simulink model "DCmotor_EMD4ETI22_Simulink_baseModel_lecture19_PEC"  (R2022a)
settings: Solver=FixedStepAuto  StartTime=0.0  StopTime=15  FixedStep=0.001  RelTol=1e-3
values from neighbouring files (symbols this model uses):
  i0 = 0    [DCmotor_InputData_baseModel_lecture19.m]    (also in DCmotor_InputData_baseModel_lecture19_PEC.m; DCmotor_InputData_baseModel_lecture19_PEC_Supply.m)
  Jeq = Inertia + Inertia_Load    [DCmotor_InputData_baseModel_lecture19.m]    (also in DCmotor_InputData_baseModel_lecture19_PEC.m = 2 * J; DCmotor_InputData_baseModel_lecture19_PEC_Supply.m = 2 * J; DCmotor_TransferFunctions_baseModel_lecture19.m)
  k_d = 0    [DCmotor_InputData_baseModel_lecture19.m]    (also in DCmotor_InputData_baseModel_lecture19_PEC.m = ViscousDamping; DCmotor_InputData_baseModel_lecture19_PEC_Supply.m = ViscousDamping; DCmotor_TransferFunctions_baseModel_lecture19.m)
  kE = Data{11, 5 + 3 * (motorID-1)}    [DCmotor_InputData_baseModel_lecture19.m]    (also in DCmotor_InputData_baseModel_lecture19_PEC.m; DCmotor_InputData_baseModel_lecture19_PEC_Supply.m; DCmotor_TransferFunctions_baseModel_lecture19.m)
  kT = Data{12, 5 + 3 * (motorID-1)}    [DCmotor_InputData_baseModel_lecture19.m]    (also in DCmotor_InputData_baseModel_lecture19_PEC.m = kE; DCmotor_InputData_baseModel_lecture19_PEC_Supply.m = kE; DCmotor_TransferFunctions_baseModel_lecture19.m)
  La = La * 10^-3    [DCmotor_InputData_baseModel_lecture19.m]    (also in DCmotor_InputData_baseModel_lecture19_PEC.m; DCmotor_InputData_baseModel_lecture19_PEC_Supply.m; DCmotor_TransferFunctions_baseModel_lecture19.m)
  pos0 = 0    [DCmotor_InputData_baseModel_lecture19.m]    (also in DCmotor_InputData_baseModel_lecture19_PEC.m; DCmotor_InputData_baseModel_lecture19_PEC_Supply.m)
  Ra_20 = Ra    [DCmotor_InputData_baseModel_lecture19.m]    (also in DCmotor_InputData_baseModel_lecture19_PEC.m; DCmotor_InputData_baseModel_lecture19_PEC_Supply.m; DCmotor_TransferFunctions_baseModel_lecture19.m)
  T_triang = 1/f_triang    (= 0.0002)    [DCmotor_InputData_baseModel_lecture19_PEC.m]    (also in DCmotor_InputData_baseModel_lecture19_PEC_Supply.m)
  V_DC = 1.5 * Voltage    [DCmotor_InputData_baseModel_lecture19_PEC.m]    (also in DCmotor_InputData_baseModel_lecture19_PEC_Supply.m)
  Voltage = Data{5, 5 + 3 * (motorID-1)}    [DCmotor_InputData_baseModel_lecture19.m]    (also in DCmotor_InputData_baseModel_lecture19_PEC.m; DCmotor_InputData_baseModel_lecture19_PEC_Supply.m; DCmotor_TransferFunctions_baseModel_lecture19.m)
  w0 = 0    [DCmotor_InputData_baseModel_lecture19.m]    (also in DCmotor_InputData_baseModel_lecture19_PEC.m; DCmotor_InputData_baseModel_lecture19_PEC_Supply.m)
libraries: simulink x1
settings Model: Creator=lucap  LastModifiedBy=lucap

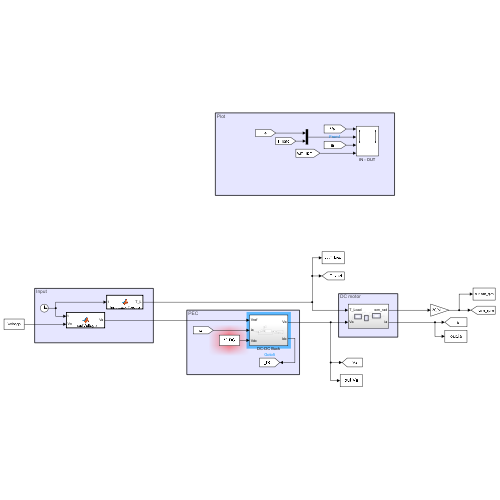
[thumbnail: Simulink's stored preview of the top-level diagram]
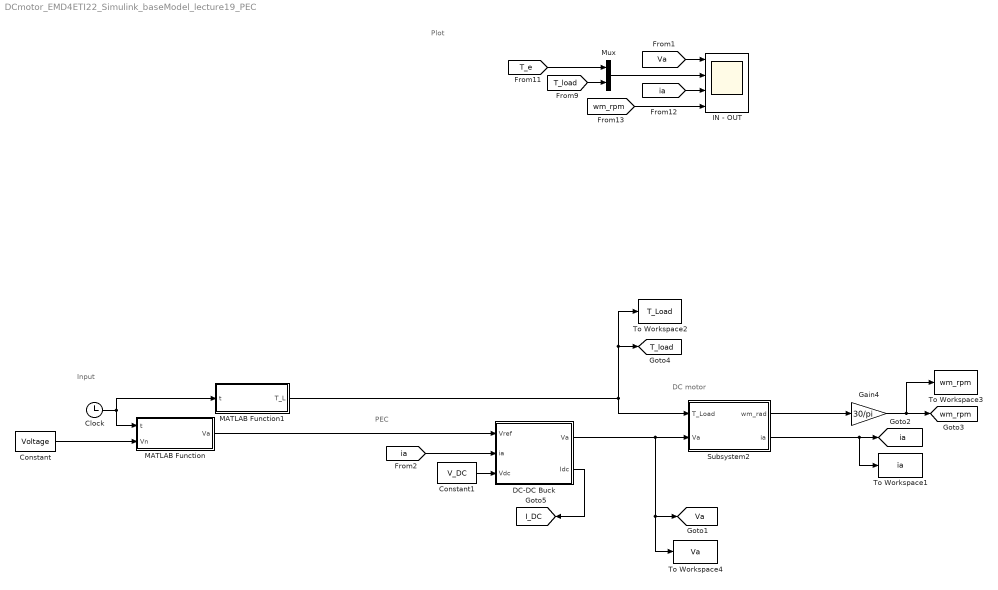
== system DCmotor_EMD4ETI22_Simulink_baseModel_lecture19_PEC ==
  note: PEC
  note: DC motor
  note: Plot
  note: Input
  Clock : Clock
  Constant : Constant  Value=Voltage
  Constant1 : Constant  Value=V_DC
  DC-DC Buck : Subsystem
  Gain4 : Gain  Gain=30/pi
  IN - OUT : Scope  NumInputPorts=4
  MATLAB Function : MATLAB Function  TreatAsAtomicUnit=on
  MATLAB Function1 : MATLAB Function  TreatAsAtomicUnit=on
  Mux : Mux  Inputs=2
  Subsystem2 : Subsystem
  To Workspace1 : ToWorkspace  VariableName=ia  SaveFormat=Structure With Time  SampleTime=-1
  To Workspace2 : ToWorkspace  VariableName=T_Load  SaveFormat=Structure With Time  SampleTime=-1
  To Workspace3 : ToWorkspace  VariableName=wm_rpm  SaveFormat=Structure With Time  SampleTime=-1
  To Workspace4 : ToWorkspace  VariableName=Va  SaveFormat=Structure With Time  SampleTime=-1
  tag scope: I_DC=global, T_load=global, Va=global, ia=global, wm_rpm=global
  wires:
  Subsystem2/1(wm_rad) -> Gain4/1
  Clock/1 -> MATLAB Function/1(t), MATLAB Function1/1(t)
  [T_e] -> Mux/1
  MATLAB Function1/1(T_L) -> [T_load], To Workspace2/1, Subsystem2/1(T_Load)
  Subsystem2/2(ia) -> To Workspace1/1, [ia]
  Gain4/1 -> To Workspace3/1, [wm_rpm]
  [T_load] -> Mux/2
  [Va] -> IN - OUT/1
  [wm_rpm] -> IN - OUT/4
  Constant/1 -> MATLAB Function/2(Vn)
  Mux/1 -> IN - OUT/2
  [ia] -> IN - OUT/3
  DC-DC Buck/1(Va) -> To Workspace4/1, [Va], Subsystem2/2(Va)
  MATLAB Function/1(Va) -> DC-DC Buck/1(Vref)
  [ia] -> DC-DC Buck/2(ia)
  Constant1/1 -> DC-DC Buck/3(Vdc)
  DC-DC Buck/2(Idc) -> [I_DC]

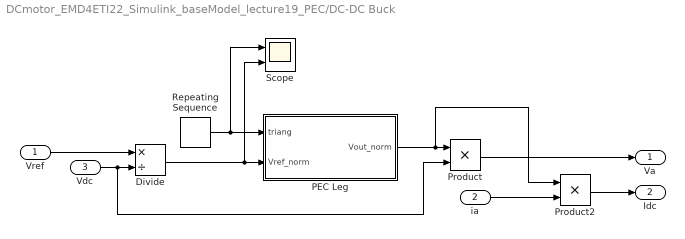
== system DCmotor_EMD4ETI22_Simulink_baseModel_lecture19_PEC/DC-DC Buck ==
  Vref : Inport
  ia : Inport  Port=2
  Vdc : Inport  Port=3
  Divide : Product  Inputs=*/
  PEC Leg : MATLAB Function  TreatAsAtomicUnit=on
  Product : Product
  Product2 : Product
  Repeating Sequence : simulink/Sources/Repeating Sequence  rep_seq_t=[0 T_triang/2 T_triang]  rep_seq_y=[0 1 0]
  Scope : Scope  NumInputPorts=2
  Va : Outport
  Idc : Outport  Port=2
  wires:
  ia/1 -> Product2/2
  Product/1 -> Va/1
  Product2/1 -> Idc/1
  Repeating Sequence/1 -> Scope/1, PEC Leg/1(triang)
  Divide/1 -> Scope/2, PEC Leg/2(Vref_norm)
  Vref/1 -> Divide/1
  Vdc/1 -> Product/2, Divide/2
  PEC Leg/1(Vout_norm) -> Product2/1, Product/1

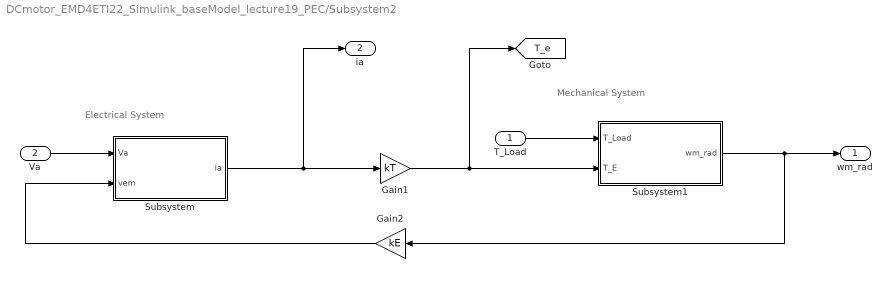
== system DCmotor_EMD4ETI22_Simulink_baseModel_lecture19_PEC/Subsystem2 ==
  note: Mechanical System
  note: Electrical System
  T_Load : Inport
  Va : Inport  Port=2
  Gain1 : Gain  Gain=kT
  Gain2 : Gain  Gain=kE
  Subsystem : Subsystem
  Subsystem1 : Subsystem
  wm_rad : Outport
  ia : Outport  Port=2
  tag scope: T_e=global
  wires:
  Subsystem/1(ia) -> Gain1/1, ia/1
  Subsystem1/1(wm_rad) -> wm_rad/1, Gain2/1
  Gain2/1 -> Subsystem/2(vem)
  Va/1 -> Subsystem/1(Va)
  Gain1/1 -> Subsystem1/2(T_E), [T_e]
  T_Load/1 -> Subsystem1/1(T_Load)

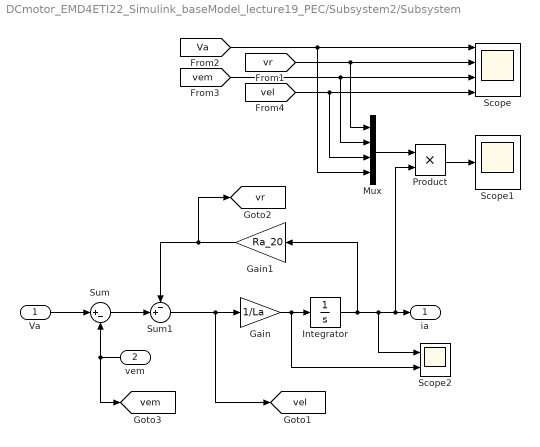
== system DCmotor_EMD4ETI22_Simulink_baseModel_lecture19_PEC/Subsystem2/Subsystem ==
  Va : Inport
  vem : Inport  Port=2
  Gain : Gain  Gain=1/La
  Gain1 : Gain  Gain=Ra_20
  Integrator : Integrator  InitialCondition=i0
  Mux : Mux
  Product : Product
  Scope : Scope  NumInputPorts=4
  Scope1 : Scope
  Scope2 : Scope  NumInputPorts=2
  Sum : Sum  Inputs=|+-
  Sum1 : Sum  Inputs=-+|
  ia : Outport
  tag scope: vel=global, vem=global, vr=global
  wires:
  Gain/1 -> Scope2/2, Integrator/1
  Va/1 -> Sum/1
  Sum/1 -> Sum1/2
  Sum1/1 -> [vel], Gain/1
  Integrator/1 -> Gain1/1, Scope2/1, Product/2, ia/1
  vem/1 -> [vem], Sum/2
  Gain1/1 -> [vr], Sum1/1
  [Va] -> Mux/4, Scope/1
  [vr] -> Mux/1, Scope/2
  [vem] -> Mux/2, Scope/3
  [vel] -> Mux/3, Scope/4
  Mux/1 -> Product/1
  Product/1 -> Scope1/1

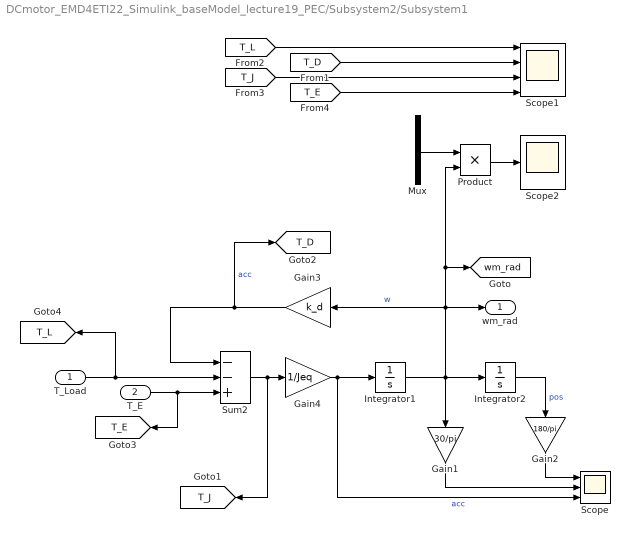
== system DCmotor_EMD4ETI22_Simulink_baseModel_lecture19_PEC/Subsystem2/Subsystem1 ==
  T_Load : Inport
  T_E : Inport  Port=2
  Gain1 : Gain  Gain=30/pi
  Gain2 : Gain  Gain=180/pi
  Gain3 : Gain  Gain=k_d
  Gain4 : Gain  Gain=1/Jeq
  Integrator1 : Integrator  InitialCondition=w0
  Integrator2 : Integrator  InitialCondition=pos0  WrapState=on  WrappedStateUpperValue=2*pi  WrappedStateLowerValue=0
  Mux : Mux
  Product : Product
  Scope : Scope  NumInputPorts=3
  Scope1 : Scope  NumInputPorts=4
  Scope2 : Scope
  Sum2 : Sum  Inputs=--+
  wm_rad : Outport
  tag scope: T_D=global, T_E=global, T_J=global, T_L=global, wm_rad=global
  wires:
  Sum2/1 -> [T_J], Gain4/1
  Gain4/1 -> Integrator1/1, Scope/3  "acc"
  Integrator1/1 -> Gain1/1, Integrator2/1, Gain3/1, Product/2, [wm_rad], wm_rad/1  "w"
  Gain1/1 -> Scope/2
  Integrator2/1 -> Gain2/1  "pos"
  Gain2/1 -> Scope/1
  T_E/1 -> [T_E], Sum2/3
  T_Load/1 -> [T_L], Sum2/2
  Gain3/1 -> [T_D], Sum2/1  "acc"
  [T_L] -> Scope1/1
  [T_E] -> Scope1/4
  [T_D] -> Scope1/2
  [T_J] -> Scope1/3
  Product/1 -> Scope2/1
  Mux/1 -> Product/1

== matlab function DCmotor_EMD4ETI22_Simulink_baseModel_lecture19_PEC/MATLAB Function ==
  data: t input; Va output; Vn input
function Va = InputVoltage(t, Vn)

t_on = 0.5;
volt_second = 7;

if (t < t_on)
    Va = 0;

elseif (t > t_on) 
    Va = volt_second * (t - t_on);

else
    Va = 0;

end

if Va > Vn 
    Va = Vn;

end

== matlab function DCmotor_EMD4ETI22_Simulink_baseModel_lecture19_PEC/DC-DC Buck/PEC Leg ==
  data: triang input; Vref_norm input; Vout_norm output
function Vout_norm = PEC_Leg(triang, Vref_norm)

if Vref_norm > triang
    Vout_norm = 1;
else
    Vout_norm = 0;
end

== matlab function DCmotor_EMD4ETI22_Simulink_baseModel_lecture19_PEC/MATLAB Function1 ==
  data: t input; T_L output
function T_L = InputLoadTorque(t)
t_load = 8;

if (t < t_load)
    T_L = 0;

elseif (t > t_load) 
    T_L = 1.5;

else
    T_L = 0;

end
